simulink model "gm_parallel_phase_voltages_per_switching_state_6_vnl"  (R2022a)
settings: Solver=FixedStepDiscrete  StartTime=0.0  StopTime=10.0  RelTol=1e-3
undefined symbols (not defined in the file or in its folder): f_c, Rt, u_dc
libraries: hdlmdlgenlib x82, simulink x6, hdlsllib x2
(part 2 of 7)

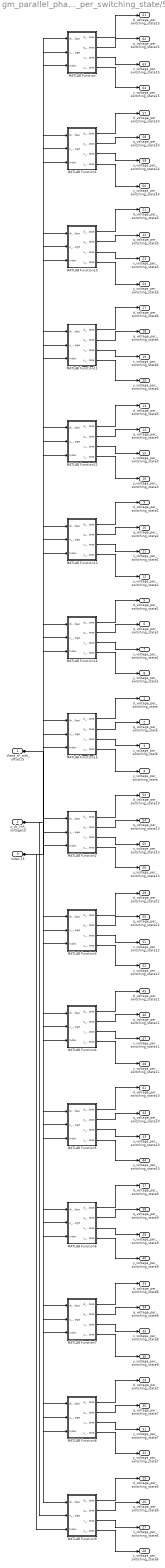
== system gm_parallel_phase_voltages_per_switching_state_6_vnl/Phase_voltages_per_switching_state/Subsystem ==
  theta_el_with_offset15 : Inport  OutDataTypeStr=single  PortDimensions=1  SampleTime=1e-08
  u_dc_link_voltage15 : Inport  Port=2  OutDataTypeStr=single  PortDimensions=1  SampleTime=1e-08
  Index 15 : Inport  Port=3  OutDataTypeStr=int32  PortDimensions=1  SampleTime=1e-08
  MATLAB Function : Subsystem
  MATLAB Function1 : Subsystem
  MATLAB Function10 : Subsystem
  MATLAB Function11 : Subsystem
  MATLAB Function12 : Subsystem
  MATLAB Function13 : Subsystem
  MATLAB Function14 : Subsystem
  MATLAB Function15 : Subsystem
  MATLAB Function2 : Subsystem
  MATLAB Function3 : Subsystem
  MATLAB Function4 : Subsystem
  MATLAB Function5 : Subsystem
  MATLAB Function6 : Subsystem
  MATLAB Function7 : Subsystem
  MATLAB Function8 : Subsystem
  MATLAB Function9 : Subsystem
  d_voltage_per_switching_state : Outport  SampleTime=1e-08
  q_voltage_per_switching_state : Outport  Port=2  SampleTime=1e-08
  x_voltage_per_switching_state : Outport  Port=3  SampleTime=1e-08
  y_voltage_per_switching_state : Outport  Port=4  SampleTime=1e-08
  d_voltage_per_switching_state1 : Outport  Port=5  SampleTime=1e-08
  q_voltage_per_switching_state1 : Outport  Port=6  SampleTime=1e-08
  x_voltage_per_switching_state1 : Outport  Port=7  SampleTime=1e-08
  y_voltage_per_switching_state1 : Outport  Port=8  SampleTime=1e-08
  d_voltage_per_switching_state2 : Outport  Port=9  SampleTime=1e-08
  q_voltage_per_switching_state2 : Outport  Port=10  SampleTime=1e-08
  x_voltage_per_switching_state2 : Outport  Port=11  SampleTime=1e-08
  y_voltage_per_switching_state2 : Outport  Port=12  SampleTime=1e-08
  d_voltage_per_switching_state3 : Outport  Port=13  SampleTime=1e-08
  q_voltage_per_switching_state3 : Outport  Port=14  SampleTime=1e-08
  x_voltage_per_switching_state3 : Outport  Port=15  SampleTime=1e-08
  y_voltage_per_switching_state3 : Outport  Port=16  SampleTime=1e-08
  d_voltage_per_switching_state4 : Outport  Port=17  SampleTime=1e-08
  q_voltage_per_switching_state4 : Outport  Port=18  SampleTime=1e-08
  x_voltage_per_switching_state4 : Outport  Port=19  SampleTime=1e-08
  y_voltage_per_switching_state4 : Outport  Port=20  SampleTime=1e-08
  d_voltage_per_switching_state5 : Outport  Port=21  SampleTime=1e-08
  q_voltage_per_switching_state5 : Outport  Port=22  SampleTime=1e-08
  x_voltage_per_switching_state5 : Outport  Port=23  SampleTime=1e-08
  y_voltage_per_switching_state5 : Outport  Port=24  SampleTime=1e-08
  d_voltage_per_switching_state6 : Outport  Port=25  SampleTime=1e-08
  q_voltage_per_switching_state6 : Outport  Port=26  SampleTime=1e-08
  x_voltage_per_switching_state6 : Outport  Port=27  SampleTime=1e-08
  y_voltage_per_switching_state6 : Outport  Port=28  SampleTime=1e-08
  d_voltage_per_switching_state7 : Outport  Port=29  SampleTime=1e-08
  q_voltage_per_switching_state7 : Outport  Port=30  SampleTime=1e-08
  x_voltage_per_switching_state7 : Outport  Port=31  SampleTime=1e-08
  y_voltage_per_switching_state7 : Outport  Port=32  SampleTime=1e-08
  d_voltage_per_switching_state8 : Outport  Port=33  SampleTime=1e-08
  q_voltage_per_switching_state8 : Outport  Port=34  SampleTime=1e-08
  x_voltage_per_switching_state8 : Outport  Port=35  SampleTime=1e-08
  y_voltage_per_switching_state8 : Outport  Port=36  SampleTime=1e-08
  d_voltage_per_switching_state9 : Outport  Port=37  SampleTime=1e-08
  q_voltage_per_switching_state9 : Outport  Port=38  SampleTime=1e-08
  x_voltage_per_switching_state9 : Outport  Port=39  SampleTime=1e-08
  y_voltage_per_switching_state9 : Outport  Port=40  SampleTime=1e-08
  d_voltage_per_switching_state10 : Outport  Port=41  SampleTime=1e-08
  q_voltage_per_switching_state10 : Outport  Port=42  SampleTime=1e-08
  x_voltage_per_switching_state10 : Outport  Port=43  SampleTime=1e-08
  y_voltage_per_switching_state10 : Outport  Port=44  SampleTime=1e-08
  d_voltage_per_switching_state11 : Outport  Port=45  SampleTime=1e-08
  q_voltage_per_switching_state11 : Outport  Port=46  SampleTime=1e-08
  x_voltage_per_switching_state11 : Outport  Port=47  SampleTime=1e-08
  y_voltage_per_switching_state11 : Outport  Port=48  SampleTime=1e-08
  d_voltage_per_switching_state12 : Outport  Port=49  SampleTime=1e-08
  q_voltage_per_switching_state12 : Outport  Port=50  SampleTime=1e-08
  x_voltage_per_switching_state12 : Outport  Port=51  SampleTime=1e-08
  y_voltage_per_switching_state12 : Outport  Port=52  SampleTime=1e-08
  d_voltage_per_switching_state13 : Outport  Port=53  SampleTime=1e-08
  q_voltage_per_switching_state13 : Outport  Port=54  SampleTime=1e-08
  x_voltage_per_switching_state13 : Outport  Port=55  SampleTime=1e-08
  y_voltage_per_switching_state13 : Outport  Port=56  SampleTime=1e-08
  d_voltage_per_switching_state14 : Outport  Port=57  SampleTime=1e-08
  q_voltage_per_switching_state14 : Outport  Port=58  SampleTime=1e-08
  x_voltage_per_switching_state14 : Outport  Port=59  SampleTime=1e-08
  y_voltage_per_switching_state14 : Outport  Port=60  SampleTime=1e-08
  d_voltage_per_switching_state15 : Outport  Port=61  SampleTime=1e-08
  q_voltage_per_switching_state15 : Outport  Port=62  SampleTime=1e-08
  x_voltage_per_switching_state15 : Outport  Port=63  SampleTime=1e-08
  y_voltage_per_switching_state15 : Outport  Port=64  SampleTime=1e-08
  wires:
  Index 15/1 -> MATLAB Function/3(Index), MATLAB Function1/3(Index), MATLAB Function10/3(Index), MATLAB Function11/3(Index), MATLAB Function12/3(Index), MATLAB Function13/3(Index), MATLAB Function14/3(Index), MATLAB Function15/3(Index), MATLAB Function2/3(Index), MATLAB Function3/3(Index), MATLAB Function4/3(Index), MATLAB Function5/3(Index), MATLAB Function6/3(Index), MATLAB Function7/3(Index), MATLAB Function8/3(Index), MATLAB Function9/3(Index)
  u_dc_link_voltage15/1 -> MATLAB Function/2(u_dc_link_voltage), MATLAB Function1/2(u_dc_link_voltage), MATLAB Function10/2(u_dc_link_voltage), MATLAB Function11/2(u_dc_link_voltage), MATLAB Function12/2(u_dc_link_voltage), MATLAB Function13/2(u_dc_link_voltage), MATLAB Function14/2(u_dc_link_voltage), MATLAB Function15/2(u_dc_link_voltage), MATLAB Function2/2(u_dc_link_voltage), MATLAB Function3/2(u_dc_link_voltage), MATLAB Function4/2(u_dc_link_voltage), MATLAB Function5/2(u_dc_link_voltage), MATLAB Function6/2(u_dc_link_voltage), MATLAB Function7/2(u_dc_link_voltage), MATLAB Function8/2(u_dc_link_voltage), MATLAB Function9/2(u_dc_link_voltage)
  theta_el_with_offset15/1 -> MATLAB Function/1(theta_el_with_offset), MATLAB Function1/1(theta_el_with_offset), MATLAB Function10/1(theta_el_with_offset), MATLAB Function11/1(theta_el_with_offset), MATLAB Function12/1(theta_el_with_offset), MATLAB Function13/1(theta_el_with_offset), MATLAB Function14/1(theta_el_with_offset), MATLAB Function15/1(theta_el_with_offset), MATLAB Function2/1(theta_el_with_offset), MATLAB Function3/1(theta_el_with_offset), MATLAB Function4/1(theta_el_with_offset), MATLAB Function5/1(theta_el_with_offset), MATLAB Function6/1(theta_el_with_offset), MATLAB Function7/1(theta_el_with_offset), MATLAB Function8/1(theta_el_with_offset), MATLAB Function9/1(theta_el_with_offset)
  MATLAB Function9/4(y_voltage_per_switching_state) -> y_voltage_per_switching_state6/1
  MATLAB Function9/3(x_voltage_per_switching_state) -> x_voltage_per_switching_state6/1
  MATLAB Function9/2(q_voltage_per_switching_state) -> q_voltage_per_switching_state6/1
  MATLAB Function9/1(d_voltage_per_switching_state) -> d_voltage_per_switching_state6/1
  MATLAB Function8/4(y_voltage_per_switching_state) -> y_voltage_per_switching_state7/1
  MATLAB Function8/3(x_voltage_per_switching_state) -> x_voltage_per_switching_state7/1
  MATLAB Function8/2(q_voltage_per_switching_state) -> q_voltage_per_switching_state7/1
  MATLAB Function8/1(d_voltage_per_switching_state) -> d_voltage_per_switching_state7/1
  MATLAB Function7/4(y_voltage_per_switching_state) -> y_voltage_per_switching_state8/1
  MATLAB Function7/3(x_voltage_per_switching_state) -> x_voltage_per_switching_state8/1
  MATLAB Function7/2(q_voltage_per_switching_state) -> q_voltage_per_switching_state8/1
  MATLAB Function7/1(d_voltage_per_switching_state) -> d_voltage_per_switching_state8/1
  MATLAB Function6/4(y_voltage_per_switching_state) -> y_voltage_per_switching_state9/1
  MATLAB Function6/3(x_voltage_per_switching_state) -> x_voltage_per_switching_state9/1
  MATLAB Function6/2(q_voltage_per_switching_state) -> q_voltage_per_switching_state9/1
  MATLAB Function6/1(d_voltage_per_switching_state) -> d_voltage_per_switching_state9/1
  MATLAB Function5/4(y_voltage_per_switching_state) -> y_voltage_per_switching_state10/1
  MATLAB Function5/3(x_voltage_per_switching_state) -> x_voltage_per_switching_state10/1
  MATLAB Function5/2(q_voltage_per_switching_state) -> q_voltage_per_switching_state10/1
  MATLAB Function5/1(d_voltage_per_switching_state) -> d_voltage_per_switching_state10/1
  MATLAB Function4/4(y_voltage_per_switching_state) -> y_voltage_per_switching_state11/1
  MATLAB Function4/3(x_voltage_per_switching_state) -> x_voltage_per_switching_state11/1
  MATLAB Function4/2(q_voltage_per_switching_state) -> q_voltage_per_switching_state11/1
  MATLAB Function4/1(d_voltage_per_switching_state) -> d_voltage_per_switching_state11/1
  MATLAB Function3/4(y_voltage_per_switching_state) -> y_voltage_per_switching_state12/1
  MATLAB Function3/3(x_voltage_per_switching_state) -> x_voltage_per_switching_state12/1
  MATLAB Function3/2(q_voltage_per_switching_state) -> q_voltage_per_switching_state12/1
  MATLAB Function3/1(d_voltage_per_switching_state) -> d_voltage_per_switching_state12/1
  MATLAB Function2/4(y_voltage_per_switching_state) -> y_voltage_per_switching_state13/1
  MATLAB Function2/3(x_voltage_per_switching_state) -> x_voltage_per_switching_state13/1
  MATLAB Function2/2(q_voltage_per_switching_state) -> q_voltage_per_switching_state13/1
  MATLAB Function2/1(d_voltage_per_switching_state) -> d_voltage_per_switching_state13/1
  MATLAB Function15/4(y_voltage_per_switching_state) -> y_voltage_per_switching_state/1
  MATLAB Function15/3(x_voltage_per_switching_state) -> x_voltage_per_switching_state/1
  MATLAB Function15/2(q_voltage_per_switching_state) -> q_voltage_per_switching_state/1
  MATLAB Function15/1(d_voltage_per_switching_state) -> d_voltage_per_switching_state/1
  MATLAB Function14/4(y_voltage_per_switching_state) -> y_voltage_per_switching_state1/1
  MATLAB Function14/3(x_voltage_per_switching_state) -> x_voltage_per_switching_state1/1
  MATLAB Function14/2(q_voltage_per_switching_state) -> q_voltage_per_switching_state1/1
  MATLAB Function14/1(d_voltage_per_switching_state) -> d_voltage_per_switching_state1/1
  MATLAB Function13/4(y_voltage_per_switching_state) -> y_voltage_per_switching_state2/1
  MATLAB Function13/3(x_voltage_per_switching_state) -> x_voltage_per_switching_state2/1
  MATLAB Function13/2(q_voltage_per_switching_state) -> q_voltage_per_switching_state2/1
  MATLAB Function13/1(d_voltage_per_switching_state) -> d_voltage_per_switching_state2/1
  MATLAB Function12/4(y_voltage_per_switching_state) -> y_voltage_per_switching_state3/1
  MATLAB Function12/3(x_voltage_per_switching_state) -> x_voltage_per_switching_state3/1
  MATLAB Function12/2(q_voltage_per_switching_state) -> q_voltage_per_switching_state3/1
  MATLAB Function12/1(d_voltage_per_switching_state) -> d_voltage_per_switching_state3/1
  MATLAB Function11/4(y_voltage_per_switching_state) -> y_voltage_per_switching_state4/1
  MATLAB Function11/3(x_voltage_per_switching_state) -> x_voltage_per_switching_state4/1
  MATLAB Function11/2(q_voltage_per_switching_state) -> q_voltage_per_switching_state4/1
  MATLAB Function11/1(d_voltage_per_switching_state) -> d_voltage_per_switching_state4/1
  MATLAB Function10/4(y_voltage_per_switching_state) -> y_voltage_per_switching_state5/1
  MATLAB Function10/3(x_voltage_per_switching_state) -> x_voltage_per_switching_state5/1
  MATLAB Function10/2(q_voltage_per_switching_state) -> q_voltage_per_switching_state5/1
  MATLAB Function10/1(d_voltage_per_switching_state) -> d_voltage_per_switching_state5/1
  MATLAB Function1/4(y_voltage_per_switching_state) -> y_voltage_per_switching_state14/1
  MATLAB Function1/3(x_voltage_per_switching_state) -> x_voltage_per_switching_state14/1
  MATLAB Function1/2(q_voltage_per_switching_state) -> q_voltage_per_switching_state14/1
  MATLAB Function1/1(d_voltage_per_switching_state) -> d_voltage_per_switching_state14/1
  MATLAB Function/4(y_voltage_per_switching_state) -> y_voltage_per_switching_state15/1
  MATLAB Function/3(x_voltage_per_switching_state) -> x_voltage_per_switching_state15/1
  MATLAB Function/2(q_voltage_per_switching_state) -> q_voltage_per_switching_state15/1
  MATLAB Function/1(d_voltage_per_switching_state) -> d_voltage_per_switching_state15/1

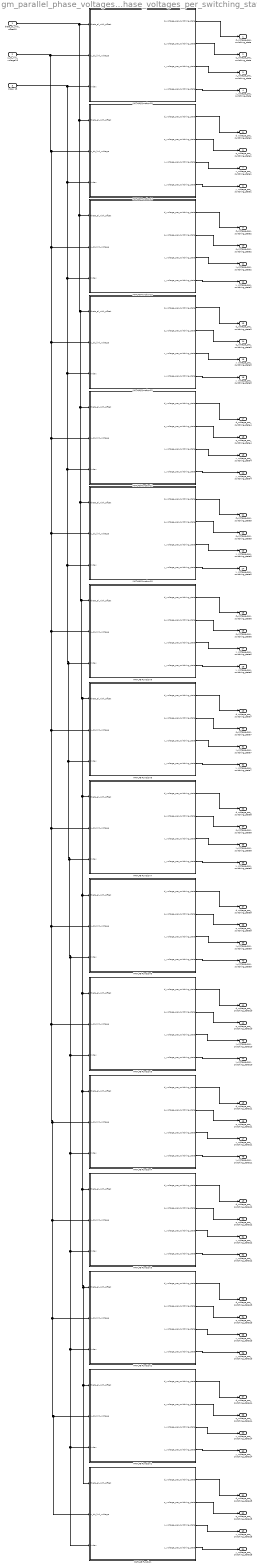
== system gm_parallel_phase_voltages_per_switching_state_6_vnl/Phase_voltages_per_switching_state_vnl/Subsystem ==
  theta_el_with_offset15 : Inport
  u_dc_link_voltage15 : Inport  Port=2
  Index 15 : Inport  Port=3
  MATLAB Function : MATLAB Function  TreatAsAtomicUnit=on
  MATLAB Function1 : MATLAB Function  TreatAsAtomicUnit=on
  MATLAB Function10 : MATLAB Function  TreatAsAtomicUnit=on
  MATLAB Function11 : MATLAB Function  TreatAsAtomicUnit=on
  MATLAB Function12 : MATLAB Function  TreatAsAtomicUnit=on
  MATLAB Function13 : MATLAB Function  TreatAsAtomicUnit=on
  MATLAB Function14 : MATLAB Function  TreatAsAtomicUnit=on
  MATLAB Function15 : MATLAB Function  TreatAsAtomicUnit=on
  MATLAB Function2 : MATLAB Function  TreatAsAtomicUnit=on
  MATLAB Function3 : MATLAB Function  TreatAsAtomicUnit=on
  MATLAB Function4 : MATLAB Function  TreatAsAtomicUnit=on
  MATLAB Function5 : MATLAB Function  TreatAsAtomicUnit=on
  MATLAB Function6 : MATLAB Function  TreatAsAtomicUnit=on
  MATLAB Function7 : MATLAB Function  TreatAsAtomicUnit=on
  MATLAB Function8 : MATLAB Function  TreatAsAtomicUnit=on
  MATLAB Function9 : MATLAB Function  TreatAsAtomicUnit=on
  d_voltage_per_switching_state : Outport
  q_voltage_per_switching_state : Outport  Port=2
  x_voltage_per_switching_state : Outport  Port=3
  y_voltage_per_switching_state : Outport  Port=4
  d_voltage_per_switching_state1 : Outport  Port=5
  q_voltage_per_switching_state1 : Outport  Port=6
  x_voltage_per_switching_state1 : Outport  Port=7
  y_voltage_per_switching_state1 : Outport  Port=8
  d_voltage_per_switching_state2 : Outport  Port=9
  q_voltage_per_switching_state2 : Outport  Port=10
  x_voltage_per_switching_state2 : Outport  Port=11
  y_voltage_per_switching_state2 : Outport  Port=12
  d_voltage_per_switching_state3 : Outport  Port=13
  q_voltage_per_switching_state3 : Outport  Port=14
  x_voltage_per_switching_state3 : Outport  Port=15
  y_voltage_per_switching_state3 : Outport  Port=16
  d_voltage_per_switching_state4 : Outport  Port=17
  q_voltage_per_switching_state4 : Outport  Port=18
  x_voltage_per_switching_state4 : Outport  Port=19
  y_voltage_per_switching_state4 : Outport  Port=20
  d_voltage_per_switching_state5 : Outport  Port=21
  q_voltage_per_switching_state5 : Outport  Port=22
  x_voltage_per_switching_state5 : Outport  Port=23
  y_voltage_per_switching_state5 : Outport  Port=24
  d_voltage_per_switching_state6 : Outport  Port=25
  q_voltage_per_switching_state6 : Outport  Port=26
  x_voltage_per_switching_state6 : Outport  Port=27
  y_voltage_per_switching_state6 : Outport  Port=28
  d_voltage_per_switching_state7 : Outport  Port=29
  q_voltage_per_switching_state7 : Outport  Port=30
  x_voltage_per_switching_state7 : Outport  Port=31
  y_voltage_per_switching_state7 : Outport  Port=32
  d_voltage_per_switching_state8 : Outport  Port=33
  q_voltage_per_switching_state8 : Outport  Port=34
  x_voltage_per_switching_state8 : Outport  Port=35
  y_voltage_per_switching_state8 : Outport  Port=36
  d_voltage_per_switching_state9 : Outport  Port=37
  q_voltage_per_switching_state9 : Outport  Port=38
  x_voltage_per_switching_state9 : Outport  Port=39
  y_voltage_per_switching_state9 : Outport  Port=40
  d_voltage_per_switching_state10 : Outport  Port=41
  q_voltage_per_switching_state10 : Outport  Port=42
  x_voltage_per_switching_state10 : Outport  Port=43
  y_voltage_per_switching_state10 : Outport  Port=44
  d_voltage_per_switching_state11 : Outport  Port=45
  q_voltage_per_switching_state11 : Outport  Port=46
  x_voltage_per_switching_state11 : Outport  Port=47
  y_voltage_per_switching_state11 : Outport  Port=48
  d_voltage_per_switching_state12 : Outport  Port=49
  q_voltage_per_switching_state12 : Outport  Port=50
  x_voltage_per_switching_state12 : Outport  Port=51
  y_voltage_per_switching_state12 : Outport  Port=52
  d_voltage_per_switching_state13 : Outport  Port=53
  q_voltage_per_switching_state13 : Outport  Port=54
  x_voltage_per_switching_state13 : Outport  Port=55
  y_voltage_per_switching_state13 : Outport  Port=56
  d_voltage_per_switching_state14 : Outport  Port=57
  q_voltage_per_switching_state14 : Outport  Port=58
  x_voltage_per_switching_state14 : Outport  Port=59
  y_voltage_per_switching_state14 : Outport  Port=60
  d_voltage_per_switching_state15 : Outport  Port=61
  q_voltage_per_switching_state15 : Outport  Port=62
  x_voltage_per_switching_state15 : Outport  Port=63
  y_voltage_per_switching_state15 : Outport  Port=64
  wires:
  MATLAB Function2/4(y_voltage_per_switching_state) -> y_voltage_per_switching_state13/1
  MATLAB Function2/3(x_voltage_per_switching_state) -> x_voltage_per_switching_state13/1
  MATLAB Function5/4(y_voltage_per_switching_state) -> y_voltage_per_switching_state10/1
  MATLAB Function5/1(d_voltage_per_switching_state) -> d_voltage_per_switching_state10/1
  MATLAB Function5/2(q_voltage_per_switching_state) -> q_voltage_per_switching_state10/1
  MATLAB Function7/3(x_voltage_per_switching_state) -> x_voltage_per_switching_state8/1
  MATLAB Function7/2(q_voltage_per_switching_state) -> q_voltage_per_switching_state8/1
  MATLAB Function7/4(y_voltage_per_switching_state) -> y_voltage_per_switching_state8/1
  MATLAB Function7/1(d_voltage_per_switching_state) -> d_voltage_per_switching_state8/1
  MATLAB Function9/4(y_voltage_per_switching_state) -> y_voltage_per_switching_state6/1
  MATLAB Function9/1(d_voltage_per_switching_state) -> d_voltage_per_switching_state6/1
  MATLAB Function9/2(q_voltage_per_switching_state) -> q_voltage_per_switching_state6/1
  MATLAB Function9/3(x_voltage_per_switching_state) -> x_voltage_per_switching_state6/1
  MATLAB Function1/3(x_voltage_per_switching_state) -> x_voltage_per_switching_state14/1
  MATLAB Function1/2(q_voltage_per_switching_state) -> q_voltage_per_switching_state14/1
  Index 15/1 -> MATLAB Function14/3(Index), MATLAB Function13/3(Index), MATLAB Function12/3(Index), MATLAB Function11/3(Index), MATLAB Function9/3(Index), MATLAB Function7/3(Index), MATLAB Function6/3(Index), MATLAB Function5/3(Index), MATLAB Function4/3(Index), MATLAB Function3/3(Index), MATLAB Function2/3(Index), MATLAB Function1/3(Index), MATLAB Function/3(Index), MATLAB Function8/3(Index), MATLAB Function10/3(Index), MATLAB Function15/3(Index)
  MATLAB Function14/2(q_voltage_per_switching_state) -> q_voltage_per_switching_state1/1
  MATLAB Function14/1(d_voltage_per_switching_state) -> d_voltage_per_switching_state1/1
  MATLAB Function14/3(x_voltage_per_switching_state) -> x_voltage_per_switching_state1/1
  MATLAB Function2/2(q_voltage_per_switching_state) -> q_voltage_per_switching_state13/1
  MATLAB Function14/4(y_voltage_per_switching_state) -> y_voltage_per_switching_state1/1
  u_dc_link_voltage15/1 -> MATLAB Function15/2(u_dc_link_voltage), MATLAB Function14/2(u_dc_link_voltage), MATLAB Function13/2(u_dc_link_voltage), MATLAB Function12/2(u_dc_link_voltage), MATLAB Function11/2(u_dc_link_voltage), MATLAB Function10/2(u_dc_link_voltage), MATLAB Function9/2(u_dc_link_voltage), MATLAB Function8/2(u_dc_link_voltage), MATLAB Function7/2(u_dc_link_voltage), MATLAB Function6/2(u_dc_link_voltage), MATLAB Function5/2(u_dc_link_voltage), MATLAB Function4/2(u_dc_link_voltage), MATLAB Function3/2(u_dc_link_voltage), MATLAB Function2/2(u_dc_link_voltage), MATLAB Function1/2(u_dc_link_voltage), MATLAB Function/2(u_dc_link_voltage)
  MATLAB Function/2(q_voltage_per_switching_state) -> q_voltage_per_switching_state15/1
  MATLAB Function/4(y_voltage_per_switching_state) -> y_voltage_per_switching_state15/1
  MATLAB Function15/3(x_voltage_per_switching_state) -> x_voltage_per_switching_state/1
  MATLAB Function15/4(y_voltage_per_switching_state) -> y_voltage_per_switching_state/1
  MATLAB Function15/1(d_voltage_per_switching_state) -> d_voltage_per_switching_state/1
  MATLAB Function6/4(y_voltage_per_switching_state) -> y_voltage_per_switching_state9/1
  MATLAB Function6/1(d_voltage_per_switching_state) -> d_voltage_per_switching_state9/1
  MATLAB Function6/3(x_voltage_per_switching_state) -> x_voltage_per_switching_state9/1
  MATLAB Function5/3(x_voltage_per_switching_state) -> x_voltage_per_switching_state10/1
  MATLAB Function6/2(q_voltage_per_switching_state) -> q_voltage_per_switching_state9/1
  MATLAB Function4/2(q_voltage_per_switching_state) -> q_voltage_per_switching_state11/1
  MATLAB Function12/2(q_voltage_per_switching_state) -> q_voltage_per_switching_state3/1
  MATLAB Function1/1(d_voltage_per_switching_state) -> d_voltage_per_switching_state14/1
  MATLAB Function1/4(y_voltage_per_switching_state) -> y_voltage_per_switching_state14/1
  MATLAB Function13/3(x_voltage_per_switching_state) -> x_voltage_per_switching_state2/1
  MATLAB Function13/1(d_voltage_per_switching_state) -> d_voltage_per_switching_state2/1
  MATLAB Function8/4(y_voltage_per_switching_state) -> y_voltage_per_switching_state7/1
  MATLAB Function13/4(y_voltage_per_switching_state) -> y_voltage_per_switching_state2/1
  MATLAB Function3/3(x_voltage_per_switching_state) -> x_voltage_per_switching_state12/1
  MATLAB Function4/4(y_voltage_per_switching_state) -> y_voltage_per_switching_state11/1
  MATLAB Function10/2(q_voltage_per_switching_state) -> q_voltage_per_switching_state5/1
  MATLAB Function10/1(d_voltage_per_switching_state) -> d_voltage_per_switching_state5/1
  MATLAB Function13/2(q_voltage_per_switching_state) -> q_voltage_per_switching_state2/1
  MATLAB Function/3(x_voltage_per_switching_state) -> x_voltage_per_switching_state15/1
  MATLAB Function12/4(y_voltage_per_switching_state) -> y_voltage_per_switching_state3/1
  MATLAB Function2/1(d_voltage_per_switching_state) -> d_voltage_per_switching_state13/1
  MATLAB Function12/1(d_voltage_per_switching_state) -> d_voltage_per_switching_state3/1
  MATLAB Function11/2(q_voltage_per_switching_state) -> q_voltage_per_switching_state4/1
  MATLAB Function4/3(x_voltage_per_switching_state) -> x_voltage_per_switching_state11/1
  MATLAB Function10/4(y_voltage_per_switching_state) -> y_voltage_per_switching_state5/1
  MATLAB Function11/3(x_voltage_per_switching_state) -> x_voltage_per_switching_state4/1
  MATLAB Function/1(d_voltage_per_switching_state) -> d_voltage_per_switching_state15/1
  MATLAB Function8/3(x_voltage_per_switching_state) -> x_voltage_per_switching_state7/1
  MATLAB Function15/2(q_voltage_per_switching_state) -> q_voltage_per_switching_state/1
  MATLAB Function12/3(x_voltage_per_switching_state) -> x_voltage_per_switching_state3/1
  theta_el_with_offset15/1 -> MATLAB Function15/1(theta_el_with_offset), MATLAB Function14/1(theta_el_with_offset), MATLAB Function13/1(theta_el_with_offset), MATLAB Function12/1(theta_el_with_offset), MATLAB Function11/1(theta_el_with_offset), MATLAB Function10/1(theta_el_with_offset), MATLAB Function9/1(theta_el_with_offset), MATLAB Function8/1(theta_el_with_offset), MATLAB Function7/1(theta_el_with_offset), MATLAB Function6/1(theta_el_with_offset), MATLAB Function5/1(theta_el_with_offset), MATLAB Function4/1(theta_el_with_offset), MATLAB Function3/1(theta_el_with_offset), MATLAB Function2/1(theta_el_with_offset), MATLAB Function1/1(theta_el_with_offset), MATLAB Function/1(theta_el_with_offset)
  MATLAB Function11/1(d_voltage_per_switching_state) -> d_voltage_per_switching_state4/1
  MATLAB Function3/1(d_voltage_per_switching_state) -> d_voltage_per_switching_state12/1
  MATLAB Function8/2(q_voltage_per_switching_state) -> q_voltage_per_switching_state7/1
  MATLAB Function8/1(d_voltage_per_switching_state) -> d_voltage_per_switching_state7/1
  MATLAB Function10/3(x_voltage_per_switching_state) -> x_voltage_per_switching_state5/1
  MATLAB Function3/4(y_voltage_per_switching_state) -> y_voltage_per_switching_state12/1
  MATLAB Function3/2(q_voltage_per_switching_state) -> q_voltage_per_switching_state12/1
  MATLAB Function11/4(y_voltage_per_switching_state) -> y_voltage_per_switching_state4/1
  MATLAB Function4/1(d_voltage_per_switching_state) -> d_voltage_per_switching_state11/1

== system gm_parallel_phase_voltages_per_switching_state_6_vnl/Phase_voltages_per_switching_state/Detect Rise Positive/Positive ==
  u : Inport  OutDataTypeStr=boolean  SampleTime=1e-08
  Compare : RelationalOperator  Operator=>  OutDataTypeStr=boolean  ZeroCross=off
  Constant : Constant  DisableCoverage=on  Value=0  OutDataTypeStr=Inherit: Inherit via back propagation  SampleTime=-1  PreserveConstantTs=on
  y : Outport  SampleTime=1e-08
  wires:
  u/1 -> Compare/1
  Constant/1 -> Compare/2
  Compare/1 -> y/1

== system gm_parallel_phase_voltages_per_switching_state_6_vnl/Phase_voltages_per_switching_state/Detect Rise Positive1/Positive ==
  u : Inport  OutDataTypeStr=boolean  SampleTime=1e-08
  Compare : RelationalOperator  Operator=>  OutDataTypeStr=boolean  ZeroCross=off
  Constant : Constant  DisableCoverage=on  Value=0  OutDataTypeStr=Inherit: Inherit via back propagation  SampleTime=-1  PreserveConstantTs=on
  y : Outport  SampleTime=1e-08
  wires:
  u/1 -> Compare/1
  Constant/1 -> Compare/2
  Compare/1 -> y/1

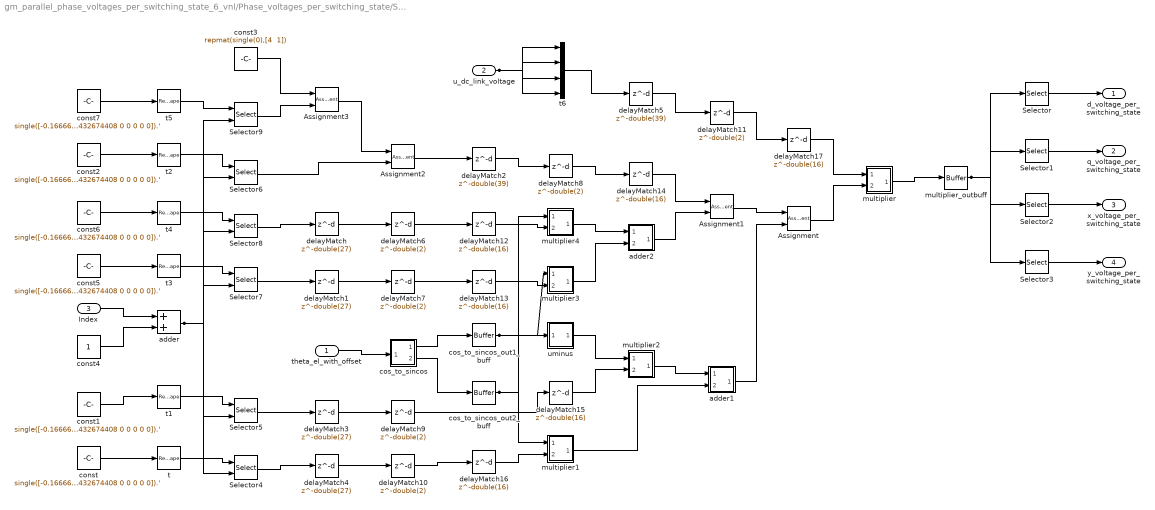
== system gm_parallel_phase_voltages_per_switching_state_6_vnl/Phase_voltages_per_switching_state/Subsystem/MATLAB Function ==
  theta_el_with_offset : Inport  OutDataTypeStr=single  PortDimensions=1  SampleTime=1e-08
  u_dc_link_voltage : Inport  Port=2  OutDataTypeStr=single  PortDimensions=1  SampleTime=1e-08
  Index : Inport  Port=3  OutDataTypeStr=int32  PortDimensions=1  SampleTime=1e-08
  Assignment : Assignment  NumberOfDimensions=2  SampleTime=1e-08  IndexOptions=Index vector (dialog),Index vector (dialog)  Indices=double(2),double(1)  OutputSizes=double(0),double(0)
  Assignment1 : Assignment  NumberOfDimensions=2  SampleTime=1e-08  IndexOptions=Index vector (dialog),Index vector (dialog)  Indices=double(1),double(1)  OutputSizes=double(0),double(0)
  Assignment2 : Assignment  NumberOfDimensions=2  SampleTime=1e-08  IndexOptions=Index vector (dialog),Index vector (dialog)  Indices=double(4),double(1)  OutputSizes=double(0),double(0)
  Assignment3 : Assignment  NumberOfDimensions=2  SampleTime=1e-08  IndexOptions=Index vector (dialog),Index vector (dialog)  Indices=double(3),double(1)  OutputSizes=double(0),double(0)
  Selector : Selector  NumberOfDimensions=2  SampleTime=1e-08  IndexOptions=Index vector (dialog),Index vector (dialog)  Indices=double(1),double(1)  OutputSizes=double(0),double(0)
  Selector1 : Selector  NumberOfDimensions=2  SampleTime=1e-08  IndexOptions=Index vector (dialog),Index vector (dialog)  Indices=double(2),double(1)  OutputSizes=double(0),double(0)
  Selector2 : Selector  NumberOfDimensions=2  SampleTime=1e-08  IndexOptions=Index vector (dialog),Index vector (dialog)  Indices=double(3),double(1)  OutputSizes=double(0),double(0)
  Selector3 : Selector  NumberOfDimensions=2  SampleTime=1e-08  IndexOptions=Index vector (dialog),Index vector (dialog)  Indices=double(4),double(1)  OutputSizes=double(0),double(0)
  Selector4 : Selector  NumberOfDimensions=2  SampleTime=1e-08  IndexOptions=Index vector (dialog),Index vector (port)  Indices=double(2),double(-1)  OutputSizes=double(0),double(0)
  Selector5 : Selector  NumberOfDimensions=2  SampleTime=1e-08  IndexOptions=Index vector (dialog),Index vector (port)  Indices=double(1),double(-1)  OutputSizes=double(0),double(0)
  Selector6 : Selector  NumberOfDimensions=2  SampleTime=1e-08  IndexOptions=Index vector (dialog),Index vector (port)  Indices=double(4),double(-1)  OutputSizes=double(0),double(0)
  Selector7 : Selector  NumberOfDimensions=2  SampleTime=1e-08  IndexOptions=Index vector (dialog),Index vector (port)  Indices=double(2),double(-1)  OutputSizes=double(0),double(0)
  Selector8 : Selector  NumberOfDimensions=2  SampleTime=1e-08  IndexOptions=Index vector (dialog),Index vector (port)  Indices=double(1),double(-1)  OutputSizes=double(0),double(0)
  Selector9 : Selector  NumberOfDimensions=2  SampleTime=1e-08  IndexOptions=Index vector (dialog),Index vector (port)  Indices=double(3),double(-1)  OutputSizes=double(0),double(0)
  adder : Sum  AccumDataTypeStr=int32  OutDataTypeStr=int32  RndMeth=Nearest  SaturateOnIntegerOverflow=on  SampleTime=1e-08
  adder1 : Subsystem
      mask Display: disp('NFP\nadd');
  adder2 : Subsystem
      mask Display: disp('NFP\nadd');
  const{,1..2,5..7} (6 alike) : Constant  Value=single([-0.1666666716337204 -0.28867512941360474 -0.1666666716337204 0.28867512941360474 0.1666666716337204 -0.28867512941360474 0.1666666716337204 0.28867512941360474 -0.3333333432674408 0 -0.3333333432674408 0 0 0 0 0]).'  VectorParams1D=off  OutDataTypeStr=single  SampleTime=1e-08
  const3 : Constant  Value="repmat(single(0),[4  1])"  VectorParams1D=off  OutDataTypeStr=single  SampleTime=1e-08
  const4 : Constant  VectorParams1D=off  OutDataTypeStr=int32  SampleTime=1e-08
  cos_to_sincos : Subsystem
      mask Display: disp('NFP\ntrig2');
  cos_to_sincos_out1_buff : hdlmdlgenlib/Buffer
      settings: SourceProductBaseCode=SL
  cos_to_sincos_out2_buff : hdlmdlgenlib/Buffer
      settings: SourceProductBaseCode=SL
  delayMatch{,1,3..4} (4 alike) : Delay  DelayLength=double(27)  InitialCondition=0  SampleTime=1e-08
  delayMatch{6..11} (6 alike) : Delay  DelayLength=double(2)  InitialCondition=0  SampleTime=1e-08
  delayMatch{12..17} (6 alike) : Delay  DelayLength=double(16)  InitialCondition=0  SampleTime=1e-08
  delayMatch2 : Delay  DelayLength=double(39)  InitialCondition=0  SampleTime=1e-08
  delayMatch5 : Delay  DelayLength=double(39)  InitialCondition=0  SampleTime=1e-08
  multiplier : Subsystem
      mask Display: disp('NFP\nmul');
  multiplier1 : Subsystem
      mask Display: disp('NFP\nmul');
  multiplier2 : Subsystem
      mask Display: disp('NFP\nmul');
  multiplier3 : Subsystem
      mask Display: disp('NFP\nmul');
  multiplier4 : Subsystem
      mask Display: disp('NFP\nmul');
  multiplier_outbuff : hdlmdlgenlib/Buffer
      settings: SourceProductBaseCode=SL
  t{,1..5} (6 alike) : Reshape  OutputDimensionality=Customize  OutputDimensions=[4,4]
  t6 : Mux
  uminus : Subsystem
      mask Display: disp('NFP\numinus');
  d_voltage_per_switching_state : Outport  SampleTime=1e-08  VectorParamsAs1DForOutWhenUnconnected=off
  q_voltage_per_switching_state : Outport  Port=2  SampleTime=1e-08
  x_voltage_per_switching_state : Outport  Port=3  SampleTime=1e-08
  y_voltage_per_switching_state : Outport  Port=4  SampleTime=1e-08
  wires:
  Index/1 -> adder/1
  u_dc_link_voltage/1 -> t6/1, t6/2, t6/3, t6/4
  theta_el_with_offset/1 -> cos_to_sincos/1(In1)
  delayMatch11/1 -> delayMatch17/1
  delayMatch10/1 -> delayMatch16/1
  delayMatch9/1 -> delayMatch15/1
  delayMatch8/1 -> delayMatch14/1
  delayMatch7/1 -> delayMatch13/1
  delayMatch6/1 -> delayMatch12/1
  delayMatch5/1 -> delayMatch11/1
  delayMatch4/1 -> delayMatch10/1
  delayMatch3/1 -> delayMatch9/1
  delayMatch2/1 -> delayMatch8/1
  delayMatch1/1 -> delayMatch7/1
  delayMatch/1 -> delayMatch6/1
  t6/1 -> delayMatch5/1
  Selector4/1 -> delayMatch4/1
  Selector5/1 -> delayMatch3/1
  Assignment2/1 -> delayMatch2/1
  Selector7/1 -> delayMatch1/1
  Selector8/1 -> delayMatch/1
  cos_to_sincos/2(Out2) -> cos_to_sincos_out2_buff/1
  cos_to_sincos/1(Out1) -> cos_to_sincos_out1_buff/1
  multiplier4/1(Out1) -> adder2/1(In1)
  multiplier3/1(Out1) -> adder2/2(In2)
  uminus/1(Out1) -> multiplier2/1(In1)
  adder2/1(Out1) -> Assignment1/2
  multiplier2/1(Out1) -> adder1/1(In1)
  multiplier1/1(Out1) -> adder1/2(In2)
  adder1/1(Out1) -> Assignment/2
  multiplier/1(Out1) -> multiplier_outbuff/1
  delayMatch17/1 -> multiplier/1(In1)
  const7/1 -> t5/1
  const6/1 -> t4/1
  const5/1 -> t3/1
  const2/1 -> t2/1
  const1/1 -> t1/1
  const/1 -> t/1
  t5/1 -> Selector9/1
  t4/1 -> Selector8/1
  t3/1 -> Selector7/1
  const4/1 -> adder/2
  const3/1 -> Assignment3/1
  Selector9/1 -> Assignment3/2
  t2/1 -> Selector6/1
  delayMatch12/1 -> multiplier4/2(In2)
  delayMatch13/1 -> multiplier3/2(In2)
  cos_to_sincos_out1_buff/1 -> uminus/1(In1), multiplier3/1(In1)
  t1/1 -> Selector5/1
  t/1 -> Selector4/1
  adder/1 -> Selector4/2, Selector5/2, Selector6/2, Selector7/2, Selector8/2, Selector9/2
  Assignment3/1 -> Assignment2/1
  Selector6/1 -> Assignment2/2
  delayMatch15/1 -> multiplier2/2(In2)
  cos_to_sincos_out2_buff/1 -> multiplier1/1(In1), multiplier4/1(In1)
  delayMatch16/1 -> multiplier1/2(In2)
  delayMatch14/1 -> Assignment1/1
  Assignment1/1 -> Assignment/1
  Assignment/1 -> multiplier/2(In2)
  multiplier_outbuff/1 -> Selector/1, Selector1/1, Selector2/1, Selector3/1
  Selector3/1 -> y_voltage_per_switching_state/1
  Selector2/1 -> x_voltage_per_switching_state/1
  Selector1/1 -> q_voltage_per_switching_state/1
  Selector/1 -> d_voltage_per_switching_state/1

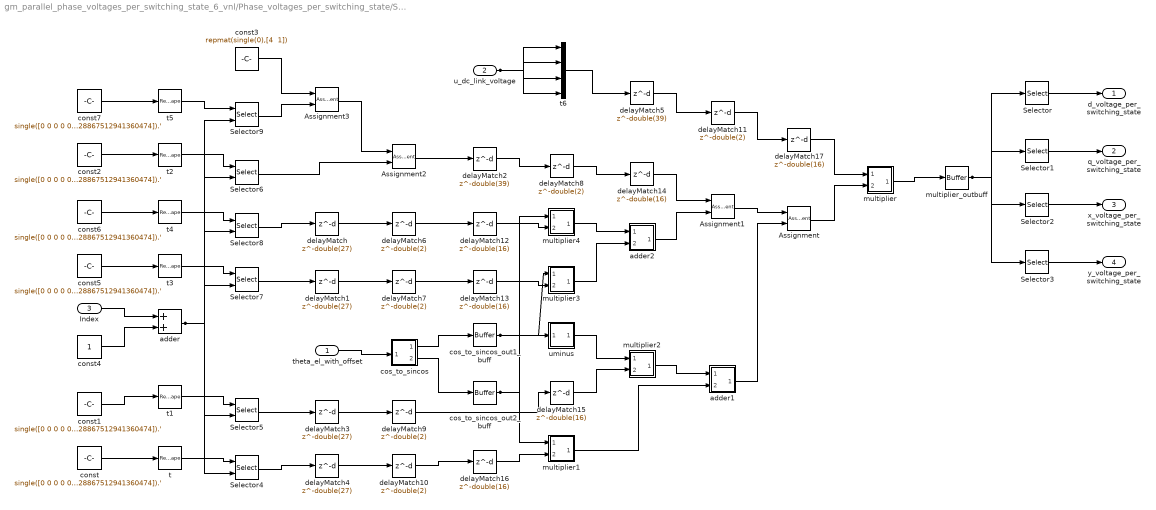
== system gm_parallel_phase_voltages_per_switching_state_6_vnl/Phase_voltages_per_switching_state/Subsystem/MATLAB Function1 ==
  theta_el_with_offset : Inport  OutDataTypeStr=single  PortDimensions=1  SampleTime=1e-08
  u_dc_link_voltage : Inport  Port=2  OutDataTypeStr=single  PortDimensions=1  SampleTime=1e-08
  Index : Inport  Port=3  OutDataTypeStr=int32  PortDimensions=1  SampleTime=1e-08
  Assignment : Assignment  NumberOfDimensions=2  SampleTime=1e-08  IndexOptions=Index vector (dialog),Index vector (dialog)  Indices=double(2),double(1)  OutputSizes=double(0),double(0)
  Assignment1 : Assignment  NumberOfDimensions=2  SampleTime=1e-08  IndexOptions=Index vector (dialog),Index vector (dialog)  Indices=double(1),double(1)  OutputSizes=double(0),double(0)
  Assignment2 : Assignment  NumberOfDimensions=2  SampleTime=1e-08  IndexOptions=Index vector (dialog),Index vector (dialog)  Indices=double(4),double(1)  OutputSizes=double(0),double(0)
  Assignment3 : Assignment  NumberOfDimensions=2  SampleTime=1e-08  IndexOptions=Index vector (dialog),Index vector (dialog)  Indices=double(3),double(1)  OutputSizes=double(0),double(0)
  Selector : Selector  NumberOfDimensions=2  SampleTime=1e-08  IndexOptions=Index vector (dialog),Index vector (dialog)  Indices=double(1),double(1)  OutputSizes=double(0),double(0)
  Selector1 : Selector  NumberOfDimensions=2  SampleTime=1e-08  IndexOptions=Index vector (dialog),Index vector (dialog)  Indices=double(2),double(1)  OutputSizes=double(0),double(0)
  Selector2 : Selector  NumberOfDimensions=2  SampleTime=1e-08  IndexOptions=Index vector (dialog),Index vector (dialog)  Indices=double(3),double(1)  OutputSizes=double(0),double(0)
  Selector3 : Selector  NumberOfDimensions=2  SampleTime=1e-08  IndexOptions=Index vector (dialog),Index vector (dialog)  Indices=double(4),double(1)  OutputSizes=double(0),double(0)
  Selector4 : Selector  NumberOfDimensions=2  SampleTime=1e-08  IndexOptions=Index vector (dialog),Index vector (port)  Indices=double(2),double(-1)  OutputSizes=double(0),double(0)
  Selector5 : Selector  NumberOfDimensions=2  SampleTime=1e-08  IndexOptions=Index vector (dialog),Index vector (port)  Indices=double(1),double(-1)  OutputSizes=double(0),double(0)
  Selector6 : Selector  NumberOfDimensions=2  SampleTime=1e-08  IndexOptions=Index vector (dialog),Index vector (port)  Indices=double(4),double(-1)  OutputSizes=double(0),double(0)
  Selector7 : Selector  NumberOfDimensions=2  SampleTime=1e-08  IndexOptions=Index vector (dialog),Index vector (port)  Indices=double(2),double(-1)  OutputSizes=double(0),double(0)
  Selector8 : Selector  NumberOfDimensions=2  SampleTime=1e-08  IndexOptions=Index vector (dialog),Index vector (port)  Indices=double(1),double(-1)  OutputSizes=double(0),double(0)
  Selector9 : Selector  NumberOfDimensions=2  SampleTime=1e-08  IndexOptions=Index vector (dialog),Index vector (port)  Indices=double(3),double(-1)  OutputSizes=double(0),double(0)
  adder : Sum  AccumDataTypeStr=int32  OutDataTypeStr=int32  RndMeth=Nearest  SaturateOnIntegerOverflow=on  SampleTime=1e-08
  adder1 : Subsystem
      mask Display: disp('NFP\nadd');
  adder2 : Subsystem
      mask Display: disp('NFP\nadd');
  const{,1..2,5..7} (6 alike) : Constant  Value=single([0 0 0 0 0.3333333432674408 0 0.3333333432674408 0 -0.1666666716337204 0.28867512941360474 -0.1666666716337204 -0.28867512941360474 0.1666666716337204 0.28867512941360474 0.1666666716337204 -0.28867512941360474]).'  VectorParams1D=off  OutDataTypeStr=single  SampleTime=1e-08
  const3 : Constant  Value="repmat(single(0),[4  1])"  VectorParams1D=off  OutDataTypeStr=single  SampleTime=1e-08
  const4 : Constant  VectorParams1D=off  OutDataTypeStr=int32  SampleTime=1e-08
  cos_to_sincos : Subsystem
      mask Display: disp('NFP\ntrig2');
  cos_to_sincos_out1_buff : hdlmdlgenlib/Buffer
      settings: SourceProductBaseCode=SL
  cos_to_sincos_out2_buff : hdlmdlgenlib/Buffer
      settings: SourceProductBaseCode=SL
  delayMatch{,1,3..4} (4 alike) : Delay  DelayLength=double(27)  InitialCondition=0  SampleTime=1e-08
  delayMatch{6..11} (6 alike) : Delay  DelayLength=double(2)  InitialCondition=0  SampleTime=1e-08
  delayMatch{12..17} (6 alike) : Delay  DelayLength=double(16)  InitialCondition=0  SampleTime=1e-08
  delayMatch2 : Delay  DelayLength=double(39)  InitialCondition=0  SampleTime=1e-08
  delayMatch5 : Delay  DelayLength=double(39)  InitialCondition=0  SampleTime=1e-08
  multiplier : Subsystem
      mask Display: disp('NFP\nmul');
  multiplier1 : Subsystem
      mask Display: disp('NFP\nmul');
  multiplier2 : Subsystem
      mask Display: disp('NFP\nmul');
  multiplier3 : Subsystem
      mask Display: disp('NFP\nmul');
  multiplier4 : Subsystem
      mask Display: disp('NFP\nmul');
  multiplier_outbuff : hdlmdlgenlib/Buffer
      settings: SourceProductBaseCode=SL
  t{,1..5} (6 alike) : Reshape  OutputDimensionality=Customize  OutputDimensions=[4,4]
  t6 : Mux
  uminus : Subsystem
      mask Display: disp('NFP\numinus');
  d_voltage_per_switching_state : Outport  SampleTime=1e-08  VectorParamsAs1DForOutWhenUnconnected=off
  q_voltage_per_switching_state : Outport  Port=2  SampleTime=1e-08
  x_voltage_per_switching_state : Outport  Port=3  SampleTime=1e-08
  y_voltage_per_switching_state : Outport  Port=4  SampleTime=1e-08
  wires:
  Index/1 -> adder/1
  u_dc_link_voltage/1 -> t6/1, t6/2, t6/3, t6/4
  theta_el_with_offset/1 -> cos_to_sincos/1(In1)
  delayMatch11/1 -> delayMatch17/1
  delayMatch10/1 -> delayMatch16/1
  delayMatch9/1 -> delayMatch15/1
  delayMatch8/1 -> delayMatch14/1
  delayMatch7/1 -> delayMatch13/1
  delayMatch6/1 -> delayMatch12/1
  delayMatch5/1 -> delayMatch11/1
  delayMatch4/1 -> delayMatch10/1
  delayMatch3/1 -> delayMatch9/1
  delayMatch2/1 -> delayMatch8/1
  delayMatch1/1 -> delayMatch7/1
  delayMatch/1 -> delayMatch6/1
  t6/1 -> delayMatch5/1
  Selector4/1 -> delayMatch4/1
  Selector5/1 -> delayMatch3/1
  Assignment2/1 -> delayMatch2/1
  Selector7/1 -> delayMatch1/1
  Selector8/1 -> delayMatch/1
  cos_to_sincos/2(Out2) -> cos_to_sincos_out2_buff/1
  cos_to_sincos/1(Out1) -> cos_to_sincos_out1_buff/1
  multiplier4/1(Out1) -> adder2/1(In1)
  multiplier3/1(Out1) -> adder2/2(In2)
  uminus/1(Out1) -> multiplier2/1(In1)
  adder2/1(Out1) -> Assignment1/2
  multiplier2/1(Out1) -> adder1/1(In1)
  multiplier1/1(Out1) -> adder1/2(In2)
  adder1/1(Out1) -> Assignment/2
  multiplier/1(Out1) -> multiplier_outbuff/1
  delayMatch17/1 -> multiplier/1(In1)
  const7/1 -> t5/1
  const6/1 -> t4/1
  const5/1 -> t3/1
  const2/1 -> t2/1
  const1/1 -> t1/1
  const/1 -> t/1
  t5/1 -> Selector9/1
  t4/1 -> Selector8/1
  t3/1 -> Selector7/1
  const4/1 -> adder/2
  const3/1 -> Assignment3/1
  Selector9/1 -> Assignment3/2
  t2/1 -> Selector6/1
  delayMatch12/1 -> multiplier4/2(In2)
  delayMatch13/1 -> multiplier3/2(In2)
  cos_to_sincos_out1_buff/1 -> uminus/1(In1), multiplier3/1(In1)
  t1/1 -> Selector5/1
  t/1 -> Selector4/1
  adder/1 -> Selector4/2, Selector5/2, Selector6/2, Selector7/2, Selector8/2, Selector9/2
  Assignment3/1 -> Assignment2/1
  Selector6/1 -> Assignment2/2
  delayMatch15/1 -> multiplier2/2(In2)
  cos_to_sincos_out2_buff/1 -> multiplier1/1(In1), multiplier4/1(In1)
  delayMatch16/1 -> multiplier1/2(In2)
  delayMatch14/1 -> Assignment1/1
  Assignment1/1 -> Assignment/1
  Assignment/1 -> multiplier/2(In2)
  multiplier_outbuff/1 -> Selector/1, Selector1/1, Selector2/1, Selector3/1
  Selector3/1 -> y_voltage_per_switching_state/1
  Selector2/1 -> x_voltage_per_switching_state/1
  Selector1/1 -> q_voltage_per_switching_state/1
  Selector/1 -> d_voltage_per_switching_state/1

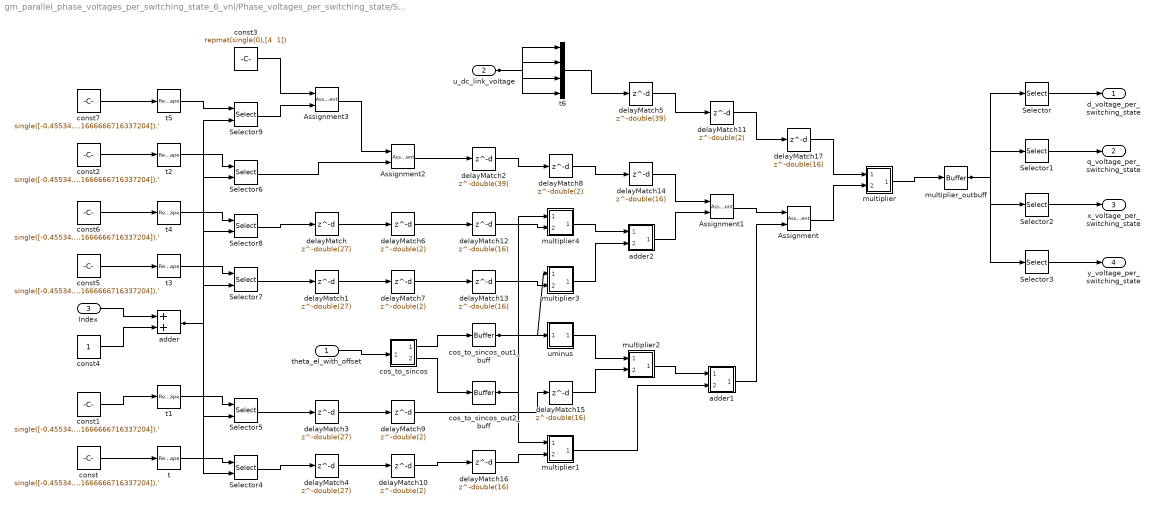
== system gm_parallel_phase_voltages_per_switching_state_6_vnl/Phase_voltages_per_switching_state/Subsystem/MATLAB Function10 ==
  theta_el_with_offset : Inport  OutDataTypeStr=single  PortDimensions=1  SampleTime=1e-08
  u_dc_link_voltage : Inport  Port=2  OutDataTypeStr=single  PortDimensions=1  SampleTime=1e-08
  Index : Inport  Port=3  OutDataTypeStr=int32  PortDimensions=1  SampleTime=1e-08
  Assignment : Assignment  NumberOfDimensions=2  SampleTime=1e-08  IndexOptions=Index vector (dialog),Index vector (dialog)  Indices=double(2),double(1)  OutputSizes=double(0),double(0)
  Assignment1 : Assignment  NumberOfDimensions=2  SampleTime=1e-08  IndexOptions=Index vector (dialog),Index vector (dialog)  Indices=double(1),double(1)  OutputSizes=double(0),double(0)
  Assignment2 : Assignment  NumberOfDimensions=2  SampleTime=1e-08  IndexOptions=Index vector (dialog),Index vector (dialog)  Indices=double(4),double(1)  OutputSizes=double(0),double(0)
  Assignment3 : Assignment  NumberOfDimensions=2  SampleTime=1e-08  IndexOptions=Index vector (dialog),Index vector (dialog)  Indices=double(3),double(1)  OutputSizes=double(0),double(0)
  Selector : Selector  NumberOfDimensions=2  SampleTime=1e-08  IndexOptions=Index vector (dialog),Index vector (dialog)  Indices=double(1),double(1)  OutputSizes=double(0),double(0)
  Selector1 : Selector  NumberOfDimensions=2  SampleTime=1e-08  IndexOptions=Index vector (dialog),Index vector (dialog)  Indices=double(2),double(1)  OutputSizes=double(0),double(0)
  Selector2 : Selector  NumberOfDimensions=2  SampleTime=1e-08  IndexOptions=Index vector (dialog),Index vector (dialog)  Indices=double(3),double(1)  OutputSizes=double(0),double(0)
  Selector3 : Selector  NumberOfDimensions=2  SampleTime=1e-08  IndexOptions=Index vector (dialog),Index vector (dialog)  Indices=double(4),double(1)  OutputSizes=double(0),double(0)
  Selector4 : Selector  NumberOfDimensions=2  SampleTime=1e-08  IndexOptions=Index vector (dialog),Index vector (port)  Indices=double(2),double(-1)  OutputSizes=double(0),double(0)
  Selector5 : Selector  NumberOfDimensions=2  SampleTime=1e-08  IndexOptions=Index vector (dialog),Index vector (port)  Indices=double(1),double(-1)  OutputSizes=double(0),double(0)
  Selector6 : Selector  NumberOfDimensions=2  SampleTime=1e-08  IndexOptions=Index vector (dialog),Index vector (port)  Indices=double(4),double(-1)  OutputSizes=double(0),double(0)
  Selector7 : Selector  NumberOfDimensions=2  SampleTime=1e-08  IndexOptions=Index vector (dialog),Index vector (port)  Indices=double(2),double(-1)  OutputSizes=double(0),double(0)
  Selector8 : Selector  NumberOfDimensions=2  SampleTime=1e-08  IndexOptions=Index vector (dialog),Index vector (port)  Indices=double(1),double(-1)  OutputSizes=double(0),double(0)
  Selector9 : Selector  NumberOfDimensions=2  SampleTime=1e-08  IndexOptions=Index vector (dialog),Index vector (port)  Indices=double(3),double(-1)  OutputSizes=double(0),double(0)
  adder : Sum  AccumDataTypeStr=int32  OutDataTypeStr=int32  RndMeth=Nearest  SaturateOnIntegerOverflow=on  SampleTime=1e-08
  adder1 : Subsystem
      mask Display: disp('NFP\nadd');
  adder2 : Subsystem
      mask Display: disp('NFP\nadd');
  const{,1..2,5..7} (6 alike) : Constant  Value=single([-0.45534181594848633 -0.12200846523046494 0.12200846523046494 0.45534181594848633 -0.12200846523046494 -0.12200846523046494 0.45534181594848633 0.45534181594848633 -0.6220084428787231 0.1666666716337204 -0.044658198952674866 0.1666666716337204 -0.28867512941360474 0.1666666716337204 0.28867512941360474 0.1666666716337204]).'  VectorParams1D=off  OutDataTypeStr=single  SampleTime=1e-08
  const3 : Constant  Value="repmat(single(0),[4  1])"  VectorParams1D=off  OutDataTypeStr=single  SampleTime=1e-08
  const4 : Constant  VectorParams1D=off  OutDataTypeStr=int32  SampleTime=1e-08
  cos_to_sincos : Subsystem
      mask Display: disp('NFP\ntrig2');
  cos_to_sincos_out1_buff : hdlmdlgenlib/Buffer
      settings: SourceProductBaseCode=SL
  cos_to_sincos_out2_buff : hdlmdlgenlib/Buffer
      settings: SourceProductBaseCode=SL
  delayMatch{,1,3..4} (4 alike) : Delay  DelayLength=double(27)  InitialCondition=0  SampleTime=1e-08
  delayMatch{6..11} (6 alike) : Delay  DelayLength=double(2)  InitialCondition=0  SampleTime=1e-08
  delayMatch{12..17} (6 alike) : Delay  DelayLength=double(16)  InitialCondition=0  SampleTime=1e-08
  delayMatch2 : Delay  DelayLength=double(39)  InitialCondition=0  SampleTime=1e-08
  delayMatch5 : Delay  DelayLength=double(39)  InitialCondition=0  SampleTime=1e-08
  multiplier : Subsystem
      mask Display: disp('NFP\nmul');
  multiplier1 : Subsystem
      mask Display: disp('NFP\nmul');
  multiplier2 : Subsystem
      mask Display: disp('NFP\nmul');
  multiplier3 : Subsystem
      mask Display: disp('NFP\nmul');
  multiplier4 : Subsystem
      mask Display: disp('NFP\nmul');
  multiplier_outbuff : hdlmdlgenlib/Buffer
      settings: SourceProductBaseCode=SL
  t{,1..5} (6 alike) : Reshape  OutputDimensionality=Customize  OutputDimensions=[4,4]
  t6 : Mux
  uminus : Subsystem
      mask Display: disp('NFP\numinus');
  d_voltage_per_switching_state : Outport  SampleTime=1e-08  VectorParamsAs1DForOutWhenUnconnected=off
  q_voltage_per_switching_state : Outport  Port=2  SampleTime=1e-08
  x_voltage_per_switching_state : Outport  Port=3  SampleTime=1e-08
  y_voltage_per_switching_state : Outport  Port=4  SampleTime=1e-08
  wires:
  Index/1 -> adder/1
  u_dc_link_voltage/1 -> t6/1, t6/2, t6/3, t6/4
  theta_el_with_offset/1 -> cos_to_sincos/1(In1)
  delayMatch11/1 -> delayMatch17/1
  delayMatch10/1 -> delayMatch16/1
  delayMatch9/1 -> delayMatch15/1
  delayMatch8/1 -> delayMatch14/1
  delayMatch7/1 -> delayMatch13/1
  delayMatch6/1 -> delayMatch12/1
  delayMatch5/1 -> delayMatch11/1
  delayMatch4/1 -> delayMatch10/1
  delayMatch3/1 -> delayMatch9/1
  delayMatch2/1 -> delayMatch8/1
  delayMatch1/1 -> delayMatch7/1
  delayMatch/1 -> delayMatch6/1
  t6/1 -> delayMatch5/1
  Selector4/1 -> delayMatch4/1
  Selector5/1 -> delayMatch3/1
  Assignment2/1 -> delayMatch2/1
  Selector7/1 -> delayMatch1/1
  Selector8/1 -> delayMatch/1
  cos_to_sincos/2(Out2) -> cos_to_sincos_out2_buff/1
  cos_to_sincos/1(Out1) -> cos_to_sincos_out1_buff/1
  multiplier4/1(Out1) -> adder2/1(In1)
  multiplier3/1(Out1) -> adder2/2(In2)
  uminus/1(Out1) -> multiplier2/1(In1)
  adder2/1(Out1) -> Assignment1/2
  multiplier2/1(Out1) -> adder1/1(In1)
  multiplier1/1(Out1) -> adder1/2(In2)
  adder1/1(Out1) -> Assignment/2
  multiplier/1(Out1) -> multiplier_outbuff/1
  delayMatch17/1 -> multiplier/1(In1)
  const7/1 -> t5/1
  const6/1 -> t4/1
  const5/1 -> t3/1
  const2/1 -> t2/1
  const1/1 -> t1/1
  const/1 -> t/1
  t5/1 -> Selector9/1
  t4/1 -> Selector8/1
  t3/1 -> Selector7/1
  const4/1 -> adder/2
  const3/1 -> Assignment3/1
  Selector9/1 -> Assignment3/2
  t2/1 -> Selector6/1
  delayMatch12/1 -> multiplier4/2(In2)
  delayMatch13/1 -> multiplier3/2(In2)
  cos_to_sincos_out1_buff/1 -> uminus/1(In1), multiplier3/1(In1)
  t1/1 -> Selector5/1
  t/1 -> Selector4/1
  adder/1 -> Selector4/2, Selector5/2, Selector6/2, Selector7/2, Selector8/2, Selector9/2
  Assignment3/1 -> Assignment2/1
  Selector6/1 -> Assignment2/2
  delayMatch15/1 -> multiplier2/2(In2)
  cos_to_sincos_out2_buff/1 -> multiplier1/1(In1), multiplier4/1(In1)
  delayMatch16/1 -> multiplier1/2(In2)
  delayMatch14/1 -> Assignment1/1
  Assignment1/1 -> Assignment/1
  Assignment/1 -> multiplier/2(In2)
  multiplier_outbuff/1 -> Selector/1, Selector1/1, Selector2/1, Selector3/1
  Selector3/1 -> y_voltage_per_switching_state/1
  Selector2/1 -> x_voltage_per_switching_state/1
  Selector1/1 -> q_voltage_per_switching_state/1
  Selector/1 -> d_voltage_per_switching_state/1
